simulink model "test_clump_unclump"  (Simulink 7.3)
settings: Solver=ode45  StartTime=0  StopTime=20  RelTol=1e-3
libraries: xbsIndex_r4 x24, isi_correlator_lib x2, xps_library x1, casper_library x1
settings Model: Creator=wjm  LastModifiedBy=wjm

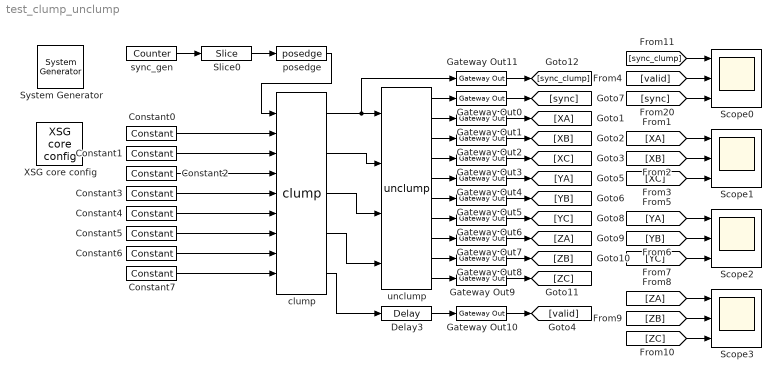
== system test_clump_unclump ==
  " System Generator" : xbsIndex_r4/ System Generator  Tag=genX  SystemSampleTime=-1  xilinxfamily=virtex5  part=xc5vsx95t  speed=-1  package=ff1136  synthesis_tool=XST  clock_wrapper=Clock Enables  directory=./test_link_mux_demux/sysgen  testbench=off  simulink_period=1  sysclk_period=5  dcm_input_clock_period=100  incr_netlist=off  trim_vbits=Everywhere in SubSystem  dbl_ovrd=According to Block Masks  core_generation=According to Block Masks  run_coregen=off  deprecated_control=off  eval_field=0  block_type=sysgen
      settings: block_version=10.1.1
  Constant0 : xbsIndex_r4/Constant  arith_type=Unsigned  const=1  n_bits=8  bin_pt=0  explicit_period=on  period=1  equ=P=C  opselect=C  inp2=PCIN>>17  opr=+  inp1=P  carry=CIN  dbl_ovrd=off  block_type=constant
      settings: block_version=10.1.1
  Constant1 : xbsIndex_r4/Constant  arith_type=Unsigned  const=2  n_bits=8  bin_pt=0  explicit_period=on  period=1  equ=P=C  opselect=C  inp2=PCIN>>17  opr=+  inp1=P  carry=CIN  dbl_ovrd=off  block_type=constant
      settings: block_version=10.1.1
  Constant2 : xbsIndex_r4/Constant  arith_type=Unsigned  const=3  n_bits=8  bin_pt=0  explicit_period=on  period=1  equ=P=C  opselect=C  inp2=PCIN>>17  opr=+  inp1=P  carry=CIN  dbl_ovrd=off  block_type=constant
      settings: block_version=10.1.1
  Constant3 : xbsIndex_r4/Constant  arith_type=Unsigned  const=4  n_bits=8  bin_pt=0  explicit_period=on  period=1  equ=P=C  opselect=C  inp2=PCIN>>17  opr=+  inp1=P  carry=CIN  dbl_ovrd=off  block_type=constant
      settings: block_version=10.1.1
  Constant4 : xbsIndex_r4/Constant  arith_type=Unsigned  const=5  n_bits=8  bin_pt=0  explicit_period=on  period=1  equ=P=C  opselect=C  inp2=PCIN>>17  opr=+  inp1=P  carry=CIN  dbl_ovrd=off  block_type=constant
      settings: block_version=10.1.1
  Constant5 : xbsIndex_r4/Constant  arith_type=Unsigned  const=6  n_bits=8  bin_pt=0  explicit_period=on  period=1  equ=P=C  opselect=C  inp2=PCIN>>17  opr=+  inp1=P  carry=CIN  dbl_ovrd=off  block_type=constant
      settings: block_version=10.1.1
  Constant6 : xbsIndex_r4/Constant  arith_type=Unsigned  const=7  n_bits=8  bin_pt=0  explicit_period=on  period=1  equ=P=C  opselect=C  inp2=PCIN>>17  opr=+  inp1=P  carry=CIN  dbl_ovrd=off  block_type=constant
      settings: block_version=10.1.1
  Constant7 : xbsIndex_r4/Constant  arith_type=Unsigned  const=8  n_bits=8  bin_pt=0  explicit_period=on  period=1  equ=P=C  opselect=C  inp2=PCIN>>17  opr=+  inp1=P  carry=CIN  dbl_ovrd=off  block_type=constant
      settings: block_version=10.1.1
  Delay3 : xbsIndex_r4/Delay  en=off  latency=1  dbl_ovrd=off  reg_retiming=off  block_type=delay
  Gateway Out{0..11} (12 alike) : xbsIndex_r4/Gateway Out  hdl_port=on  timing_constraint=None  locs_specified=off  LOCs={}  block_type=gatewayout
      settings: infoedit="Gateway out block.  Converts Xilinx fixed point inputs into ouputs of type Simulink integer, double, or fixed point.<br><br>Hardware notes:  In hardware these blocks become top level output ports or are discarded, depending on how they are configured."  block_version=11.3
  Scope{0..3} (4 alike) : Scope  NumInputPorts=3
      Scope0 settings: YMin=-5~-5~-5  YMax=5~5~5
      Scope1 settings: YMin=-5~-5~-5  YMax=5~5~5
      Scope2 settings: YMin=-5~-5~-5  YMax=5~5~5  SaveName=ScopeData2
      Scope3 settings: YMin=-5~-5~-5  YMax=5~5~5  SaveName=ScopeData3
  Slice0 : xbsIndex_r4/Slice  nbits=1  boolean_output=on  mode=Upper Bit Location + Width  bit1=-1  base1=MSB of Input  bit0=0  base0=LSB of Input  dbl_ovrd=off  block_type=slice
      settings: block_version=10.1.1
  XSG core config : xps_library/XSG core config  Tag=xps:xsg  SystemSampleTime=-1  hw_sys=ROACH:sx95t  ibob_linux=off  clk_src=sys_clk2x  iBOB_clk_src=sys_clk  BEE2_ctrl_clk_src=sys_clk  BEE2_usr_clk_src=sys_clk  ROACH_clk_src=sys_clk2x  CORR_clk_src=sys_clk  gpio_clk_io_group=iBOB:sma  gpio_clk_bit_index=0  clk_rate=200  sample_period=1  synthesis_tool=XST  mpc_type=powerpc440_ext
  clump : isi_correlator_lib/clump  SystemSampleTime=-1  latency=1
  posedge : casper_library/Misc/posedge  Tag=Rising Edge Detector  SystemSampleTime=-1
  sync_gen : xbsIndex_r4/Counter  cnt_type=Free Running  cnt_to=Inf  operation=Up  start_count=-1  cnt_by_val=1  arith_type=Unsigned  n_bits=16  bin_pt=0  load_pin=off  rst=off  en=off  explicit_period=on  period=1  dbl_ovrd=off  use_behavioral_HDL=off  implementation=Fabric  use_rpm=off  block_type=counter
  unclump : isi_correlator_lib/unclump  SystemSampleTime=-1  latency=1
  wires:
  clump/1 -> unclump/1, Gateway Out11/1
  clump/2 -> unclump/2
  clump/3 -> unclump/3
  clump/4 -> unclump/4
  clump/5 -> Delay3/1
  Constant0/1 -> clump/2
  Constant1/1 -> clump/3
  Constant2/1 -> clump/4
  Constant3/1 -> clump/5
  Constant4/1 -> clump/6
  Constant5/1 -> clump/7
  Constant6/1 -> clump/8
  Constant7/1 -> clump/9
  sync_gen/1 -> Slice0/1
  unclump/1 -> Gateway Out0/1
  unclump/2 -> Gateway Out1/1
  unclump/3 -> Gateway Out2/1
  unclump/4 -> Gateway Out3/1
  unclump/5 -> Gateway Out4/1
  unclump/6 -> Gateway Out5/1
  unclump/7 -> Gateway Out6/1
  unclump/8 -> Gateway Out7/1
  unclump/9 -> Gateway Out8/1
  unclump/10 -> Gateway Out9/1
  Delay3/1 -> Gateway Out10/1
  Gateway Out1/1 -> [XA]
  Gateway Out2/1 -> [XB]
  Gateway Out3/1 -> [XC]
  Gateway Out4/1 -> [YA]
  Gateway Out5/1 -> [YB]
  Gateway Out6/1 -> [YC]
  Gateway Out7/1 -> [ZA]
  Gateway Out8/1 -> [ZB]
  Gateway Out9/1 -> [ZC]
  Gateway Out0/1 -> [sync]
  Gateway Out10/1 -> [valid]
  [XA] -> Scope1/1
  [XB] -> Scope1/2
  [XC] -> Scope1/3
  [YA] -> Scope2/1
  [YB] -> Scope2/2
  [YC] -> Scope2/3
  [ZA] -> Scope3/1
  [ZB] -> Scope3/2
  [ZC] -> Scope3/3
  Gateway Out11/1 -> [sync_clump]
  [sync_clump] -> Scope0/1
  posedge/1 -> clump/1
  Slice0/1 -> posedge/1
  [valid] -> Scope0/2
  [sync] -> Scope0/3
